simulink model "Airship_nonlinear_dynamics_simulink"  (R2024b)
settings: Solver=ode15s  StartTime=0.0  StopTime=1000  FixedStep=0.01  MaxStep=0.01  RelTol=1e-5  AbsTol=1e-8
InitFcn:
  | Init
values from neighbouring files (symbols this model uses):
  c = 0.465    [Init.m]    (also in Nonlinear_dynamics.m = 7; init_Skyship.m = 7)
  cf = 0.1395    [Init.m]    (also in Nonlinear_dynamics.m = 3; init_Skyship.m = 3)
  CL_alpha = 5.7    [Init.m]    (also in Nonlinear_dynamics.m; init_Skyship.m)
  D = 1.6    [Init.m]    (also in Nonlinear_dynamics.m = 14; init_Skyship.m = 14)
  delta = deg2rad(10)    [Nonlinear_dynamics.m]    (also in init_Skyship.m = -15)
  delta_e = 0    [Init.m]
  delta_r = 0    [Init.m]
  etaTDF = 1    [Init.m]    (also in Nonlinear_dynamics.m = 0.6; init_Skyship.m = 0.6)
  etaTP = 0.6    [Init.m]    (also in Nonlinear_dynamics.m; init_Skyship.m)
  fProp1 = 0    [Init.m]
  fProp2 = 0    [Init.m]
  fProp_max = 20    [Init.m]
  fTDF = 4000    [Nonlinear_dynamics.m]    (also in init_Skyship.m = 0)
  fTTP = 0    [Init.m]    (also in Nonlinear_dynamics.m = 2000; init_Skyship.m)
  FVN = [5, 5, 5]    [Init.m]    (also in Nonlinear_dynamics.m = 0; init_Skyship.m = 10)
  g = 9.81    [Init.m]    (also in Nonlinear_dynamics.m; init_Skyship.m)
  I33 = eye(3)    [Init.m]    (also in Nonlinear_dynamics.m; init_Skyship.m)
  Ixx = 1.7972    [Init.m]    (also in Nonlinear_dynamics.m = 200658; init_Skyship.m = 200658)
  Ixy = 0    [Init.m]    (also in Nonlinear_dynamics.m; init_Skyship.m)
  Ixz = 0    [Init.m]    (also in Nonlinear_dynamics.m; init_Skyship.m)
  Iyy = 4.9584    [Init.m]    (also in Nonlinear_dynamics.m = 850900; init_Skyship.m = 850900)
  Iyz = 0    [Init.m]    (also in Nonlinear_dynamics.m; init_Skyship.m)
  Izz = 7.9854    [Init.m]    (also in Nonlinear_dynamics.m = 649699; init_Skyship.m = 649699)
  k1 = keta(1)    [Init.m]    (also in Nonlinear_dynamics.m; init_Skyship.m = 0.08; ketaparameters.m = 0)
  k2 = keta(2)    [Init.m]    (also in Nonlinear_dynamics.m; init_Skyship.m = 0.89; ketaparameters.m = 0)
  k_dash = keta(3)    [Init.m]    (also in Nonlinear_dynamics.m; init_Skyship.m = 0.5; ketaparameters.m = 0)
  L = 4.7    [Init.m]    (also in Nonlinear_dynamics.m = zeros(1,4); init_Skyship.m = 52)
  m = 7.31    [Init.m]    (also in Nonlinear_dynamics.m = 5942; init_Skyship.m = 5942; velocity_tf_script.m; velocity_tf_script_v2.m)
  MAF = zeros(6,6)    [Init.m]    (also in Nonlinear_dynamics.m; init_Skyship.m)
  MVN = [0.2, 10, 5]    [Init.m]    (also in Nonlinear_dynamics.m = 0; init_Skyship.m = 0.001)
  p0 = 0    [Init.m]    (also in init_Skyship.m)
  phi0 = 0    [Init.m]    (also in init_Skyship.m)
  Prop1_alpha = 0    [Init.m]
  Prop2_alpha = 0    [Init.m]
  psi0 = 0    [Init.m]    (also in init_Skyship.m)
  q0 = 0    [Init.m]    (also in init_Skyship.m)
  r0 = 0    [Init.m]    (also in init_Skyship.m)
  rGxm = [XG-XB 0 ZG-ZB]'    [Init.m]    (also in Nonlinear_dynamics.m; init_Skyship.m)
  rho_0 = 1.225    [Init.m]    (also in Nonlinear_dynamics.m; init_Skyship.m)
  rho_he = 0.175    [Init.m]
  rTDF1 = [0 0.5 0]'    [Init.m]    (also in Nonlinear_dynamics.m = [3.5 7.87 21]'; init_Skyship.m = [3.5 7.87 21]')
  rTDF2 = [0 -0.5 0]'    [Init.m]    (also in Nonlinear_dynamics.m = [3.5 -7.87 21]'; init_Skyship.m = [3.5 -7.87 21]')
  rTTP = [0 0 0]'    [Init.m]    (also in Nonlinear_dynamics.m = [0 0 20.1]'; init_Skyship.m = [0 0 20.1]')
  Sf = 0.18135    [Init.m]    (also in Nonlinear_dynamics.m = 65; init_Skyship.m = 65)
  t_s = 0.005    [Init.m]
  theta0 = 1    [Init.m]    (also in init_Skyship.m = 0)
  u0 = 0.0    (= 0)    [Init.m]    (also in init_Skyship.m; velocity_tf_script.m = 4; velocity_tf_script_v2.m = 4)
  v0 = 0.0    (= 0)    [Init.m]    (also in init_Skyship.m)
  VB = 5.97    [Init.m]    (also in Nonlinear_dynamics.m = 5153; init_Skyship.m = 4911)
  w0 = 0.0    (= 0)    [Init.m]    (also in init_Skyship.m)
  xE0 = 0    [Init.m]    (also in init_Skyship.m)
  yE0 = 0    [Init.m]    (also in init_Skyship.m)
  zE0 = -h    (= -3.7495)    [Init.m]    (also in init_Skyship.m = -100)
undefined symbols (not defined in the file or in its folder): Sim3dSensor
libraries: slpidlib x13, simulink_extras x4, sim3dcameralib x1, sim3dlib x1, uavsim3dlib x1
(part 4 of 4)

== matlab function Airship_nonlinear_dynamics_simulink/Nonlinear dynamics1 ==
  data: u input; V_dot output double size=6; v input; w input; p input; q input; r input; phi input; theta input; psi input; XE input; YE input; ZE input; MAF input
function V_dot = Nonlinear_dynamics(u, v, w, p,q,r,phi,theta, psi, XE, YE, ZE, MAF)

% u = airship(1);
% v = airship(2);
% w = airship(3);
% p = airship(4);
% q = airship(5);
% r = airship(6);
% phi  = airship(7);
% theta = airship(8);
% psi = airship(9);
% 
% XE = airship(10);
% YE = airship(11);
altitude = -ZE; %linspace(0,12000, 500); %Altitude from 0 to 12000 m

%time = = airship(17);

%% Constants
g = 9.81;
m   = 5942; % mass
VB = 5153; %volume (m^3)
S = VB^(2/3) ; %surface area (m^2)

XB = 0; %x-origin point, m (boyancy)
ZB = 0; % z-origin point, m
XG = 7; %0.0 as given in [2], m
ZG = 5.1816; %m
rGxm = [XG-XB 0 ZG-ZB]';

L = 52; %Hull length
D = 14; %Hull max diameter
R = 5.6522; % Hull cross section radius at fins (m)
b = 14.13; %Hull centre line to fin tip length
delta = 0; %Elevator deflection 5 degrees
AR = 0.54;% Aspect ratio

keta = ketaparameters(L, D, R, b, AR, delta);

 % k1 = 0.08;
 % k2 = 0.89;
 % k_dash = 0.5;
 k1 = keta(1);
 k2 = keta(2);
 k_dash = keta(3);

etaf = 0.8;     % Example: Flap effectiveness
k44 = 0.1;      % Example: Roll damping coefficient

%eta = keta(1,4);
%etad = keta(1,5);
%etaf = keta(1,6);
%k44 = keta(1,7);
%k3D = keta(1,8);

Ixx = 200658; %moment of inerta Nm2
Iyy = 850900; %moment of inerta Nm2
Izz = 649699; %moment of inerta Nm2
Ixy =0;
Ixz =0;
Iyz =0;

%% Inertial forces (N) and moments (N-m)
I33 = eye(3);
rGx = [0 -rGxm(3) rGxm(2) ; rGxm(3) 0 -rGxm(1) ; -rGxm(2) rGxm(1) 0];
J = [ Ixx, Ixy, Ixz ; Ixy, Iyy, Iyz ; Ixz, Iyz, Izz];
Mrigid = [m*I33, -m*rGx; m*rGx,  J];
g_cap = [-sin(theta), cos(theta)*sin(phi), cos(theta)*cos(phi)]';
omg = [p q r]';
omgx = [0 -omg(3) omg(2) ; omg(3) 0 -omg(1) ; -omg(2) omg(1) 0];
V = [u v w]';

tau_I = [-m*omgx*V + m*omgx*rGx*omg ; -m*rGx*omgx*V - omgx*J*omg];


%% Gravitational forces and moments

%Atmosphere model
rho_0 = 1.225; %Density at sea level in kg/m3
H = 8400; %Scale height in meters;

%alitude range
%altitude = -airship(12); %linspace(0,12000, 500); %Altitude from 0 to 12000 m

density = rho_0 *exp(-altitude / H );
rho = density;
w = m*g;
B = VB*rho*g;
FG = w*g_cap; % Weight component in body frame (N)
tau_G = [FG; rGx*FG];

%% Aerostatic forces and moments

% first three are forces along x y z
% next three are moments along x y z 
rv = [0 0 0]'; %Since body frame is established at CV, the position ...
FAS = -rho*g*VB*g_cap; %Aerostatic forces N
tau_AS = [FAS; cross(rv,FAS)]; %Aerostatic forces and moments

%% Control forces and moments
% Constants

 V_bar  = sqrt(v^2 + u^2 + w^2)+ 1e-6 ; %true airspeed in m/s
 Sf = 65; % Surface area of the fin m^2
 c= 7 ; % Chord length of the fin
 cf = 3; %Flap chord
 
 S_FE = 65; %reference surface area m^2
 %
 delta = deg2rad(10);
 %lift curve slope
 CL_alpha = 5.7; %Change as needed
 
 %theoretical effectiveness factor tau
theta_f = acos(max(-1, min(1, 2*cf/c -1)));
 tau = 1- (theta_f - sin(theta_f)) /pi;
 
 %correction factor eta_d
 eta_d = 0.8; %simplified fucntion
 %3D effectiveness value
 k3D = 1.2; %example value
 %calc DeltaCL
 
 DeltaCL = CL_alpha *tau * eta_d * k3D * delta;
 
 DeltaCD = 1.7* (cf/c)^1.38 * (Sf / S_FE) * sin(delta)^2;
 
 %Moment calcs for each fin
 numerator = -2*sin(theta_f) - sin(2*theta_f);
 denominator = 8 * (pi - theta_f + sin(theta_f));
 
 ratio = numerator/denominator;
 
 DeltaCM1_4 = ratio*DeltaCL;
 
 %Deflection anges degrees
 theta = [45, 135, 225, 315];
 
 %initialize force and moment arrays
 
 Fx = zeros(1,4);
 Fy = zeros(1,4);
 Fz = zeros(1,4);
 
 L = zeros(1,4);
 M = zeros(1,4);
 N = zeros(1,4);
 
 %calc forces and moements for each fin
 
 for i = 1:4
     %conv theta to radians
     theta_rad = deg2rad(theta(i));
 
     %calc forces
     Fx(i) = -0.5 * rho * V_bar^2 *Sf*DeltaCD;
     Fy(i) = 0.5*rho*V_bar^2*Sf*(DeltaCL *sin(theta_rad)+ DeltaCD * cos(theta_rad));
     Fz(i) = -0.5 * rho * V_bar^2 *Sf*(DeltaCL *cos(theta_rad)- DeltaCD * sin(theta_rad));
 
     L(i) = Fz(i); %Assume y_i = 1 for simplicity
     M(i) = 0.5*rho*V_bar^2*Sf*c*DeltaCM1_4;
     N(i) = Fy(i); %Assume x_i = 1 for simplicity 
 end
 
 % Totals
 TotalFx = sum(Fx);
 TotalFy = sum(Fy);
 TotalFz = sum(Fz);
 
 TotalL = sum(L);
 TotalM = sum(M);
 TotalN = sum(N);
 
 tau_C = [TotalFx TotalFy TotalFz TotalL TotalM TotalN]';

%For natural response 
%tau_C = [0 0 0 0 0 0]';

%% Airship thrust force and moments
%Duct fan
rTDF1 = [3.5 7.87 21]'; % Position of motor wrt CV gomes pg 179
rTDF2 = [3.5 -7.87 21]';
fTDF = 4000; %Thrust at sea level; N
etaTDF = 0.6;% 
FTDF1 = etaTDF * [fTDF 0 0 ]'; %Thrust force N
FTDF2 = etaTDF * [fTDF 0 0 ]';
FTDF = FTDF1+FTDF2;
MTDF1 = cross(rTDF1, FTDF1); %Moments N-m
MTDF2 = cross(rTDF2, FTDF2);
MTDF = MTDF1 + MTDF2;

%Turbo prop
rTTP = [0 0 20.1]'; % Position of motor wrt CV
fTTP = 2000;%600;
etaTP = 0.6;
FTTP = etaTP* [fTTP 0 0 ]';
MTTP = cross(rTTP, FTTP);

FT = FTTP + FTDF;
MT = MTTP + MTDF;
tau_Th = [FT; MT];

%% Estimation of added mass matrix
% MAH - added mass of airship hull
%B = VB*rho*g %Bouyancy force
m_dash = B/g;
%I_dash = sum(m_dash * (L.^2 + D^2) / 20); 
I_dash = (m_dash * (L.^2 + D^2) / 20); 

mH11 = k1*m_dash;
mH22 = k2*m_dash;
mH33 = mH22;
mH44 = 0;
mH55 = k_dash*I_dash;
mH66 = mH55;
mH = [mH11, mH22, mH33, mH44, mH55, mH66];

MAH = diag(mH); %6x6 diagonal matrix



%% Estimation of added mass matrix
% MAH - added mass of airship hull
%B = VB*rho*g %Bouyancy force
m_dash = B/g;
I_dash = sum(m_dash * (L.^2 + D^2) / 20); 

mH11 = k1*m_dash;
mH22 = k2*m_dash;
mH33 = mH22;
mH44 = 0;
mH55 = k_dash*I_dash;
mH66 = mH55;
mH = [mH11, mH22, mH33, mH44, mH55, mH66];

MAH = diag(mH); %6x6 diagonal matrix


%% MAF calcs

%{

rho_dt = 1.158;
% Define integration variable numerically (assuming integration from R to b over x)
integrand_mF22 = @(x) rho_dt * pi * (x - (R.^2./x)).^2;
mF22 = etaf * integral(integrand_mF22, R, b);

integrand_mF35 = @(x) -rho_dt * pi * x .* (x - (R.^2./x)).^2;
mF35 = etaf * integral(integrand_mF35, R, b);

integrand_mF44 = @(x) (2/pi) * k44 * rho_dt * x.^4;
mF44 = etaf * integral(integrand_mF44, R, b);

integrand_mF55 = @(x) x.^2 .* rho_dt * pi .* (x - (R.^2./x)).^2;
mF55 = etaf * integral(integrand_mF55, R, b);

mF33 = mF22;
mF26 = -mF35;
mF66 = mF55;

MAF = zeros(6,6);
MAF(2,2) = mF22;
MAF(2,6) = mF26;
MAF(3,3) = mF33;
MAF(3,5) = mF35;
MAF(4,4) = mF44;
MAF(5,5) = mF55;
MAF(6,6) = mF66;
%}
MA_rigid = (MAH+MAF);


%% Aerodynamic forces and moments
% symmetric added mass axis
% Aerodynamic forces N and moments N-m

%extract components from the syymetric added mass axis
M11 = MA_rigid(1:3, 1:3);
M12 = MA_rigid(1:3, 4:6);
M21 = MA_rigid(4:6, 1:3);
M22 = MA_rigid(4:6, 4:6);

% Calc aero forces and moments

forces_due_to_rotation = cross(omg, (M11 * V + M12 *omg));
moments_due_to_translation = cross(V, (M11*V+M12*omg));
moments_due_to_rotation = cross (omg, (M21*V + M22*omg));

%combine into aero forces and moments (sign change - to +)
tau_A_dash = [forces_due_to_rotation; moments_due_to_translation+moments_due_to_rotation];

%% Viscous forces
FVN = 0; %Viscous force
MVN = 0; %Viscous Moment

if v == 0 && w == 0
    FV = [0 0 0]';
    MV = [0 0 0]';
else
    FV = FVN*[0 (-v/sqrt(v^2 + w^2)) (-w/sqrt(v^2 +w^2)) ]';
    MV = MVN*[0 (w/sqrt(v^2 + w^2)) (-v/sqrt(v^2 +w^2)) ]';
end
tau_V = [FV; MV];

%% Return
V_dot = zeros(6,1);
%{
disp('tau_I');
disp(tau_I);
disp('tau_G');
disp(tau_G);
disp('tau_C');
disp(tau_C);
disp('tau_AS');
disp(tau_AS);
disp('tau_A_dash');
disp(tau_A_dash);
disp('tau_Th');
disp(tau_Th);
disp('tau_V');
disp(tau_V);
%}

%                                       +tau_Imp for gusts
V_dot = (MA_rigid + Mrigid) \ (tau_I + tau_G + tau_C + tau_AS + tau_A_dash + tau_Th + tau_V);


end

== matlab function Airship_nonlinear_dynamics_simulink/Airship_model1/nonlinear dynamics piecewise3/tau_C ==
  data: u input; tau_C output size=[6, 1]; v input; w input; delta_e input; delta_r input; rho input; Sf input; c input; cf input; CL_alpha input; L_hull input

function tau_C = fcn(u, v, w, delta_e, delta_r,rho, Sf, c, cf, CL_alpha, L_hull)
V_bar  = sqrt(u^2 + v^2 + w^2); % TAS m/s
S_FE   = Sf;                    % reference surface area m^2
delta_e_rad = deg2rad(delta_e);
delta_r_rad = deg2rad(delta_r);
q = 0.5 * rho * V_bar^2;
 
 %theoretical effectiveness factor tau
 theta_f = acos(2*cf/c -1);
 tau = 1- (theta_f - sin(theta_f)) /pi;
 
 %correction factor eta_d
 eta_d = 0.8; %simplified fucntion
 %3D effectiveness value
 k3D = 1.2; %example value
 %calc DeltaCL
 
 DeltaCL_elev = CL_alpha *tau * eta_d * k3D * delta_e_rad;
 DeltaCL_rud = CL_alpha *tau * eta_d * k3D * delta_r_rad;
 DeltaCD_elev = 1.7* (cf/c)^1.38 * (Sf / S_FE) * sin(delta_e_rad)^2;
 DeltaCD_rud = 1.7* (cf/c)^1.38 * (Sf / S_FE) * sin(delta_r_rad)^2; 
   %{
 %Moment calcs for each fin
 numerator = -2*sin(theta_f) - sin(2*theta_f);
 denominator = 8 * (pi - theta_f + sin(theta_f));

 ratio = numerator/denominator;

 DeltaCM1_4_elev = ratio*DeltaCL_elev;
 DeltaCM1_4_rud = ratio*DeltaCL_rud;

 %Deflection angels degrees
 theta = [90, 270, 0, 180];
  %}
 %initialize force and moment arrays
 
 Fx = zeros(1,4); %logitudinal forces
 Fy = zeros(1,4); %lateral forces
 Fz = zeros(1,4); %vertical forces
 
 L = zeros(1,4); %rolling moment
 M = zeros(1,4); %pitching moment
 N = zeros(1,4); %yawing moment
 
 %calc forces and moements for each fin
 
 for i = 1:2
 
     %calc forces
     Fx(i) = -q *Sf*DeltaCD_elev;
     Fy(i) = 0;
     Fz(i) = q*Sf*(DeltaCL_elev);
 
     L(i) = 0;
     M(i) = Fz(i)*0.5*L_hull; %assume moment arm is haf of the hull length
     N(i) = 0;
 end
 for i = 3:4
     %calc forces
     Fx(i) = -q *Sf*DeltaCD_rud;
     Fy(i) = q *Sf*(DeltaCL_rud);
     Fz(i) = 0;
 
     L(i) = 0;
     M(i) = 0;
     N(i) = Fy(i)*0.5*L_hull; %assume moment arm is haf of the hull length
 end

 % Totals
 TotalFx = sum(Fx(:));
 TotalFy = sum(Fy(:));
 TotalFz = sum(Fz(:));

 TotalL = sum(L(:));
 TotalM = sum(M(:));
 TotalN = sum(N(:));
 tau_C = [TotalFx TotalFy TotalFz TotalL TotalM TotalN]';


end
%{
function tau_C = fcn(u, v, w, delta, rho, Sf, c, cf, CL_alpha)
% fcn computes the forces and moments exerted by the elevator.
%
% Syntax:
%   tau_C = fcn(u, v, w, delta, rho, Sf, c, cf, CL_alpha)
%
% Inputs:
%   u, v, w   - Velocities in the body axes (m/s)
%   delta     - Elevator deflection (in degrees)
%   rho       - Air density (kg/m^3)
%   Sf        - Fin (or elevator) surface area (m^2)
%   c         - Chord length of the fin (m)
%   cf        - Chord length of the flap (m)
%   CL_alpha  - Lift curve slope (per radian)
%
% Outputs:
%   tau_C     - 6x1 column vector with total force and moment components:
%               [TotalFx; TotalFy; TotalFz; TotalL; TotalM; TotalN]
%
% The function computes the force generated by the elevator using a
% simplified aerodynamic model. Later, rudder contributions can be added.
%

% -------------------------------------------------
% Constants and preliminary calculations
% -------------------------------------------------
V_bar  = sqrt(u^2 + v^2 + w^2);        % true airspeed in m/s
S_FE   = Sf;                           % reference surface area m^2
delta_rad = deg2rad(delta);            % convert deflection to radians

% Deflection angles (degrees) for all 4 fins (2 elevator and 2 rudder)
theta = [45, 135, 225, 315];

% -------------------------------------------------
% Initialize force and moment arrays
% -------------------------------------------------
% Force components (assumed to be calculated for each fin/elevator)
Fx = zeros(size(theta));  % X forces (e.g., drag)
Fy = zeros(size(theta));  % Y forces (lateral - zero in symmetric case)
Fz = zeros(size(theta));  % Z forces (lift)

% Moment components for each fin/elevator
L = zeros(size(theta));  % Rolling moment about x-axis
M = zeros(size(theta));  % Pitching moment about y-axis
N = zeros(size(theta));  % Yawing moment about z-axis

% -------------------------------------------------
% Aerodynamic force calculations
% -------------------------------------------------
% Calculate dynamic pressure
q = 0.5 * rho * V_bar^2;

% Elevator lift (simplified linear model)
% Using the relation: Lift = q * S_FE * CL_alpha * delta_rad
Lift = q * S_FE * CL_alpha * delta_rad;

% For this example, we assume that all 4 fins (or elevator surfaces)
% produce identical contributions. More nuanced models would separately
% handle the contributions from elevator vs. rudder.
%
% Here we distribute the forces and moments for each surface.
for i = 1:length(theta)
    % Forces:
    % - Fx: a small fraction (e.g., 10%) of the lift is assumed to be
    %       converted to a drag force along the x-axis.
    % - Fy: no lateral force is assumed (symmetry).
    % - Fz: the full lift is assumed to act in the vertical direction.
    Fx(i) = 0.1 * Lift;
    Fy(i) = 0;
    Fz(i) = Lift;
    
    % Moments (using chord as approximate lever arms):
    % - Rolling moment (L): assumed to be 0.5 * Lift * c
    % - Pitching moment (M): assumed to be Lift * c
    % - Yawing moment (N): assumed to be 0.5 * Lift * cf
    L(i) = 0.5 * Lift * c;
    M(i) = Lift * c;
    N(i) = 0.5 * Lift * cf;
end

% -------------------------------------------------
% Consolidate the total forces and moments
% -------------------------------------------------
TotalFx = sum(Fx(:));
TotalFy = sum(Fy(:));
TotalFz = sum(Fz(:));

TotalL  = sum(L(:));
TotalM  = sum(M(:));
TotalN  = sum(N(:));

% Output: Force and moment vector as a column vector
tau_C = [TotalFx; TotalFy; TotalFz; TotalL; TotalM; TotalN];

end
%}
%{ 
%% Control forces and moments
% Constants
 V_bar  = sqrt(v^2 + u^2 + w^2) ; %true airspeed in m/s
 S_FE = Sf; %reference surface area m^2
 delta_rad = deg2rad(delta);
 
 %theoretical effectiveness factor tau
 theta_f = acos(2*cf/c -1);
 tau = 1- (theta_f - sin(theta_f)) /pi;
 
 %correction factor eta_d
 eta_d = 0.8; %simplified fucntion
 %3D effectiveness value
 k3D = 1.2; %example value
 %calc DeltaCL
 
 DeltaCL = CL_alpha *tau * eta_d * k3D * delta_rad;
 
 DeltaCD = 1.7* (cf/c)^1.38 * (Sf / S_FE) * sin(delta_rad)^2;
 
 %Moment calcs for each fin
 numerator = -2*sin(theta_f) - sin(2*theta_f);
 denominator = 8 * (pi - theta_f + sin(theta_f));
 
 ratio = numerator/denominator;
 
 DeltaCM1_4 = ratio*DeltaCL;
 
 %Deflection angels degrees
 theta = [45, 135, 225, 315];
 
 %initialize force and moment arrays
 
 Fx = zeros(1,4);
 Fy = zeros(1,4);
 Fz = zeros(1,4);
 
 L = zeros(1,4);
 M = zeros(1,4);
 N = zeros(1,4);
 
 %calc forces and moements for each fin
 
 for i = 1:4
     %conv theta to radians
     theta_rad = deg2rad(theta(i));
 
     %calc forces
     Fx(i) = -0.5 * rho * V_bar^2 *Sf*DeltaCD;
     Fy(i) = 0.5*rho*V_bar^2*Sf*(DeltaCL *sin(theta_rad)+ DeltaCD * cos(theta_rad));
     Fz(i) = -0.5 * rho * V_bar^2 *Sf*(DeltaCL *cos(theta_rad)- DeltaCD * sin(theta_rad));
 
     L(i) = Fz(i); %Assume y_i = 1 for simplicity
     M(i) = 0.5*rho*V_bar^2*Sf*c*DeltaCM1_4;
     N(i) = Fy(i); %Assume x_i = 1 for simplicity 
 end
 % Totals
 TotalFx = sum(Fx(:));
 TotalFy = sum(Fy(:));
 TotalFz = sum(Fz(:));

 TotalL = sum(L(:));
 TotalM = sum(M(:));
 TotalN = sum(N(:));
 tau_C = [TotalFx TotalFy TotalFz TotalL TotalM TotalN]';


end
%For natural response 
%tau_C = [0 0 0 0 0 0]';
%}

== matlab function Airship_nonlinear_dynamics_simulink/Airship_model1/nonlinear dynamics piecewise3/tau_G ==
  data: rho input; tau_G output size=[6, 1]; m input; g input; VB input; rGx input; g_cap input
function tau_G = fcn(rho, m, g, VB, rGx, g_cap)
%% Gravitational forces and moments
w = m*g;

FG = w*g_cap; % Weight component in body frame (N)
tau_G = [FG; rGx*FG];
end

== matlab function Airship_nonlinear_dynamics_simulink/Airship_model1/nonlinear dynamics piecewise3/tau_I ==
  data: J input; tau_I output size=[6, 1]; rGx input; p input; q input; r input; V input; omg input; m input
function tau_I = fcn(J, rGx, p, q, r, V, omg,m)
%% Inertial forces (N) and moments (N-m)
omgx = [0 -omg(3) omg(2) ; omg(3) 0 -omg(1) ; -omg(2) omg(1) 0];

tau_I = [-m*omgx*V + m*omgx*rGx*omg ; -m*rGx*omgx*V - omgx*J*omg];
end
